simulink model "SystemAnalysis"  (R2017b)
settings: Solver=VariableStepAuto  StartTime=0.0  StopTime=5  RelTol=1e-3
values from neighbouring files (symbols this model uses):
  A = [0          1                        0                0 ... (first row only)    [InvertedPendulum.m]
  B = [0; 4/(4*M+m); 0; 3/(4*M*l+m*l)]    [InvertedPendulum.m]
  C = [1 0 0 0; 0 0 1 0]    [InvertedPendulum.m]
settings Model: Creator=Daniel Ramos  LastModifiedBy=Daniel Ramos

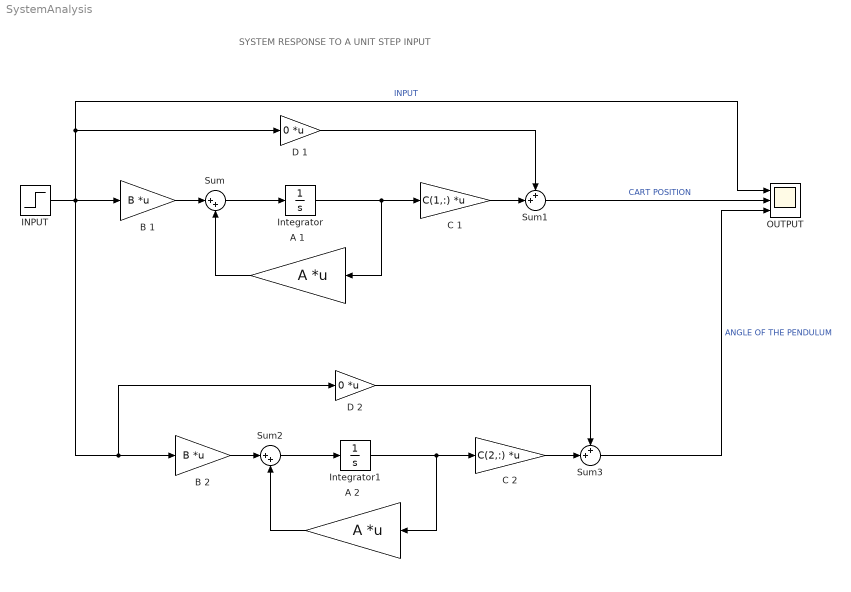
== system SystemAnalysis ==
  note: SYSTEM RESPONSE TO A UNIT STEP INPUT
  A 1 : Gain  Gain=A  Multiplication=Matrix(K*u)
  A 2 : Gain  Gain=A  Multiplication=Matrix(K*u)
  B 1 : Gain  Gain=B  Multiplication=Matrix(K*u)
  B 2 : Gain  Gain=B  Multiplication=Matrix(K*u)
  C 1 : Gain  Gain=C(1,:)  Multiplication=Matrix(K*u)
  C 2 : Gain  Gain=C(2,:)  Multiplication=Matrix(K*u)
  D 1 : Gain  Gain=0  Multiplication=Matrix(K*u)
  D 2 : Gain  Gain=0  Multiplication=Matrix(K*u)
  INPUT : Step  Time=0  SampleTime=0
  Integrator : Integrator
  Integrator1 : Integrator
  OUTPUT : Scope  NumInputPorts=3
  Sum : Sum  Inputs=|++
  Sum1 : Sum  Inputs=++|
  Sum2 : Sum  Inputs=|++
  Sum3 : Sum  Inputs=++|
  wires:
  Sum1/1 -> OUTPUT/2  "CART POSITION"
  D 1/1 -> Sum1/1
  Sum/1 -> Integrator/1
  C 1/1 -> Sum1/2
  B 1/1 -> Sum/1
  Integrator/1 -> A 1/1, C 1/1
  A 1/1 -> Sum/2
  A 2/1 -> Sum2/2
  B 2/1 -> Sum2/1
  C 2/1 -> Sum3/2
  Integrator1/1 -> A 2/1, C 2/1
  D 2/1 -> Sum3/1
  Sum3/1 -> OUTPUT/3  "ANGLE OF THE PENDULUM"
  Sum2/1 -> Integrator1/1
  INPUT/1 -> OUTPUT/1, D 1/1, B 1/1, D 2/1, B 2/1  "INPUT"
